simulink model "MSAP"  (R2023b)
settings: Solver=VariableStepAuto  StartTime=0.0  StopTime=10.0  RelTol=1e-3
undefined symbols (not defined in the file): A, F, J, L, P, PhiF, R
settings Model: Creator=lylia  LastModifiedBy=lylia

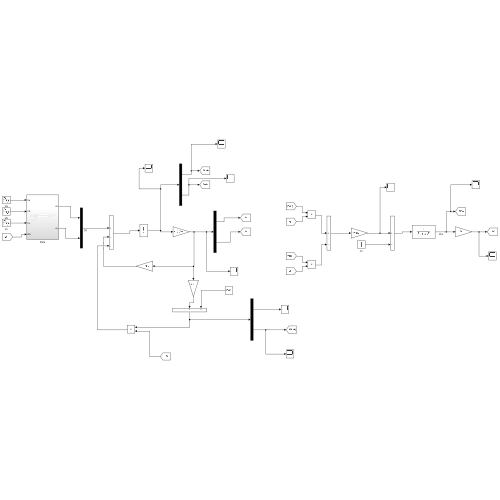
[thumbnail: Simulink's stored preview of the top-level diagram]
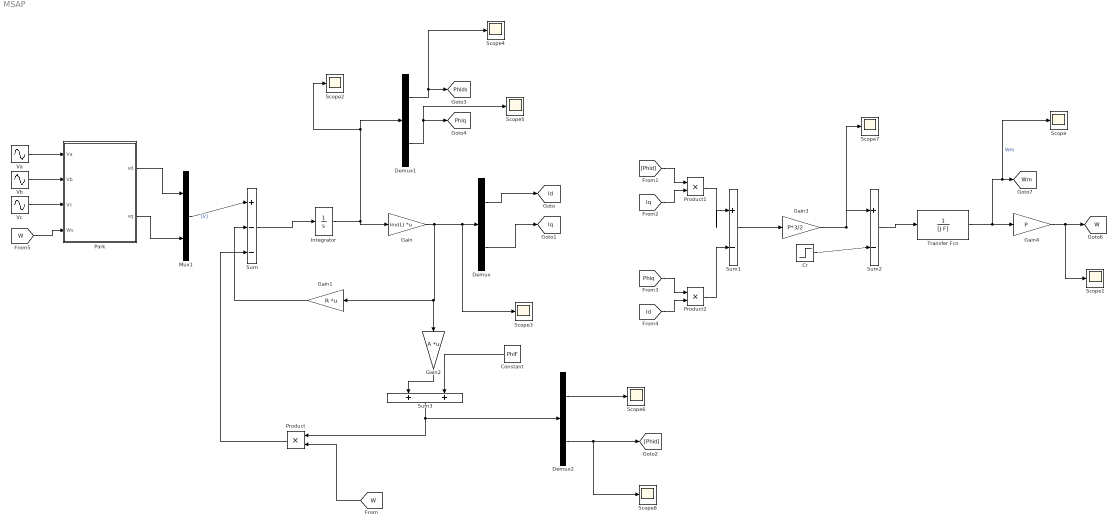
== system MSAP ==
  Constant : Constant  Value=PhiF
  Cr : Step  Time=2  Before=0.5  After=5  SampleTime=0
  Demux : Demux  Outputs=2
  Demux1 : Demux  Outputs=2
  Demux2 : Demux  Outputs=2
  Gain : Gain  Gain=inv(L)  Multiplication=Matrix(K*u)
  Gain1 : Gain  Gain=R  Multiplication=Matrix(K*u)
  Gain2 : Gain  Gain=A  Multiplication=Matrix(K*u)
  Gain3 : Gain  Gain=P*3/2
  Gain4 : Gain  Gain=P
  Integrator : Integrator
  Mux1 : Mux  Inputs=2
  Park : Subsystem
  Product : Product
  Product1 : Product
  Product2 : Product
  Scope{,1..8} (9 alike) : Scope
  Sum : Sum  Inputs=|+--
  Sum1 : Sum  Inputs=|+-
  Sum2 : Sum  Inputs=|+-
  Sum3 : Sum  Inputs=|++
  Transfer Fcn : TransferFcn  Denominator=[J F]
  Va : Sin  Amplitude=220*sqrt(2)  Frequency=2*pi*50  SampleTime=0
  Vb : Sin  Amplitude=220*sqrt(2)  Frequency=2*pi*50  Phase=-2*pi/3  SampleTime=0
  Vc : Sin  Amplitude=220*sqrt(2)  Frequency=2*pi*50  Phase=2*pi/3  SampleTime=0
  tag scope: Id=global, Iq=global, Phids=global, Phiq=global, W=global, Wm=global
  wires:
  Transfer Fcn/1 -> Scope/1, [Wm], Gain4/1  "Wm"
  [Id] -> Product2/2
  Park/2(vq) -> Mux1/2
  Vb/1 -> Park/2(Vb)
  Va/1 -> Park/1(Va)
  [W] -> Park/4(Ws)
  Integrator/1 -> Gain/1, Scope2/1, Demux1/1
  Gain1/1 -> Sum/2
  Demux/2 -> [Iq]
  Gain4/1 -> Scope1/1, [W]
  Gain/1 -> Scope3/1, Demux/1, Gain2/1, Gain1/1
  Demux1/2 -> Scope5/1, [Phiq]
  Vc/1 -> Park/3(Vc)
  [Iq] -> Product1/2
  Demux/1 -> [Id]
  Product1/1 -> Sum1/1
  Sum/1 -> Integrator/1
  Sum1/1 -> Gain3/1
  Mux1/1 -> Sum/1  "[V]"
  Gain3/1 -> Scope7/1, Sum2/1
  Product2/1 -> Sum1/2
  Demux1/1 -> Scope4/1, [Phids]
  [Phiq] -> Product2/1
  Sum2/1 -> Transfer Fcn/1
  [Phid] -> Product1/1
  Cr/1 -> Sum2/2
  Park/1(vd) -> Mux1/1
  [W] -> Product/2
  Product/1 -> Sum/3
  Gain2/1 -> Sum3/1
  Sum3/1 -> Product/1, Demux2/1
  Constant/1 -> Sum3/2
  Demux2/2 -> Scope8/1, [Phid]
  Demux2/1 -> Scope6/1

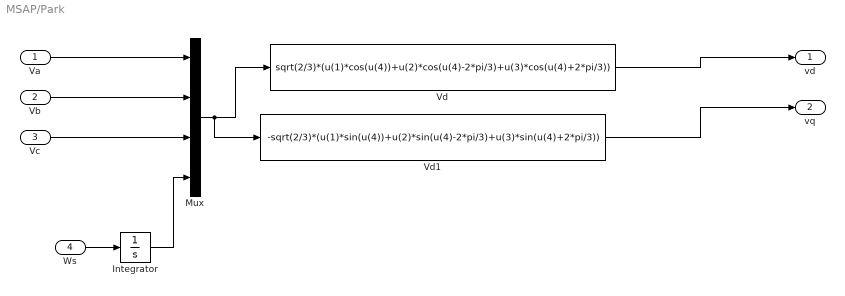
== system MSAP/Park ==
  Va : Inport
  Vb : Inport  Port=2
  Vc : Inport  Port=3
  Ws : Inport  Port=4
  Integrator : Integrator
  Mux : Mux
  Vd : Fcn  Expr=sqrt(2/3)*(u(1)*cos(u(4))+u(2)*cos(u(4)-2*pi/3)+u(3)*cos(u(4)+2*pi/3))
  Vd1 : Fcn  Expr=-sqrt(2/3)*(u(1)*sin(u(4))+u(2)*sin(u(4)-2*pi/3)+u(3)*sin(u(4)+2*pi/3))
  vd : Outport
  vq : Outport  Port=2
  wires:
  Vc/1 -> Mux/3
  Integrator/1 -> Mux/4
  Vb/1 -> Mux/2
  Vd/1 -> vd/1
  Mux/1 -> Vd1/1, Vd/1
  Va/1 -> Mux/1
  Ws/1 -> Integrator/1
  Vd1/1 -> vq/1
